simulink model "StateAttributes"  (Simulink 7.4)
settings: Solver=ode45  StartTime=0.0  StopTime=10.0  RelTol=1e-3
settings Model: Creator=dread  LastModifiedBy=dread

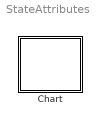
== system StateAttributes ==
  Chart : Stateflow chart

== stateflow chart Chart ==
  state State
    entry: doEntry()
    during: doDuring()
    exit: doExit()
    state SubState1 [parallel]
      settings: executionOrder=1
    state SubState2 [parallel]
      settings: executionOrder=2
  (default) -> State
  data: localVar local double; const constant double =5
  function doEntry:
    | function doEntry
    | %doEntry
  function doDuring:
    | function doDuring
    | %doDuring
  function doExit:
    | function doExit
    | %doExit
